simulink model "Lab3"  (R2023a)
settings: Solver=VariableStepAuto  StartTime=0.0  StopTime=10  RelTol=1e-3
model workspace (MAT data in the model file):
  L = 1
  g = 9.81
settings Model: Creator=Lenovo  LastModifiedBy=Lenovo

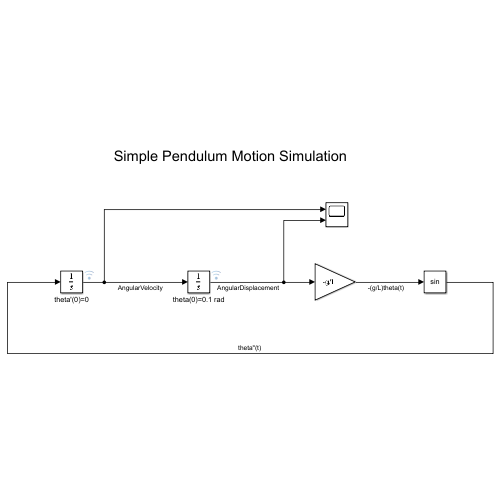
[thumbnail: Simulink's stored preview of the top-level diagram]
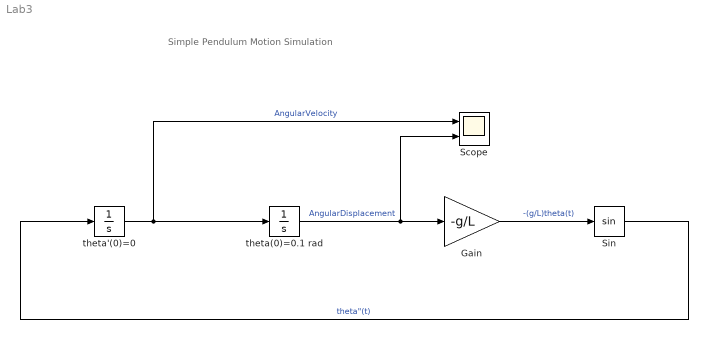
== system Lab3 ==
  note: Simple Pendulum Motion Simulation
  Gain : Gain  Gain=-g/L
  Scope : Scope  NumInputPorts=2
  Sin : Trigonometry
  theta'(0)=0 : Integrator
  theta(0)=0.1 rad : Integrator  InitialCondition=0.1
  wires:
  theta'(0)=0/1 -> Scope/1, theta(0)=0.1 rad/1  "AngularVelocity"
  theta(0)=0.1 rad/1 -> Scope/2, Gain/1  "AngularDisplacement"
  Gain/1 -> Sin/1  "-(g/L)theta(t)"
  Sin/1 -> theta'(0)=0/1  "theta\"(t)"
